simulink model "DegradationParameterBoostConverter"  (R2021a)
settings: Solver=VariableStepAuto  StartTime=0.0  StopTime=10.0  RelTol=1e-3
values from neighbouring files (symbols this model uses):
  boost_TRise_M_adjustment = -0.2    [Run_GeneratorRectifierBoostConverterInverterMotorModel.m]    (also in Run_GeneratorRectifierBoostConverterModel.m)
undefined symbols (not defined in the file or in its folder): boost_L_M_adjustment
libraries: Lib_EMTAT x3
settings Model: Creator=sfaulk  LastModifiedBy=mebell

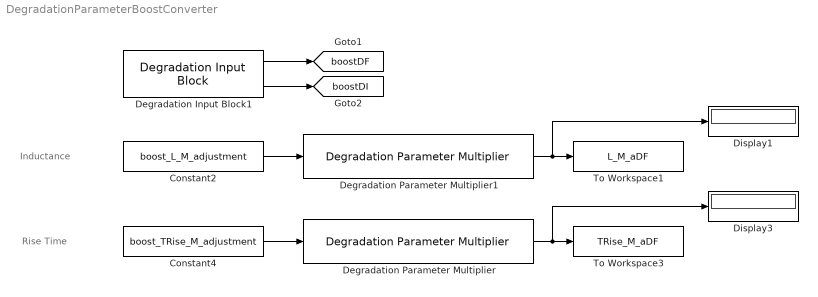
== system DegradationParameterBoostConverter ==
  note: Inductance
  note: Rise Time
  Constant2 : Constant  Value=boost_L_M_adjustment
  Constant4 : Constant  Value=boost_TRise_M_adjustment
  Degradation Input Block1 : Lib_EMTAT/Components/Physics-Based/Degradation Input Block  SystemSampleTime=-1  VariantActivationTime=update diagram  Latency=0  AutoFrameSizeCalculation=off
      settings: SourceProductName=EMTAT
  Degradation Parameter Multiplier : Lib_EMTAT/Components/Physics-Based/Degradation Parameter Multiplier  SystemSampleTime=-1  VariantActivationTime=update diagram  Latency=0  AutoFrameSizeCalculation=off
      settings: SourceProductName=EMTAT
  Degradation Parameter Multiplier1 : Lib_EMTAT/Components/Physics-Based/Degradation Parameter Multiplier  SystemSampleTime=-1  VariantActivationTime=update diagram  Latency=0  AutoFrameSizeCalculation=off
      settings: SourceProductName=EMTAT
  Display1 : Display
  Display3 : Display
  To Workspace1 : ToWorkspace  VariableName=L_M_aDF  SaveFormat=Timeseries  SampleTime=-1
      settings: Save2DSignal=2-D array (concatenate along first dimension)
  To Workspace3 : ToWorkspace  VariableName=TRise_M_aDF  SaveFormat=Timeseries  SampleTime=-1
      settings: Save2DSignal=2-D array (concatenate along first dimension)
  tag scope: boostDF=global, boostDI=global
  wires:
  Degradation Input Block1/2 -> [boostDI]
  Degradation Input Block1/1 -> [boostDF]
  Degradation Parameter Multiplier1/1 -> Display1/1, To Workspace1/1
  Constant2/1 -> Degradation Parameter Multiplier1/1
  Constant4/1 -> Degradation Parameter Multiplier/1
  Degradation Parameter Multiplier/1 -> Display3/1, To Workspace3/1
